simulink model "SVPWM_modified_working"  (R2015b)
settings: Solver=VariableStepAuto  StartTime=0.0  StopTime=0.1  RelTol=1e-3
libraries: powerlib x33, simulink x7
settings Model: Creator=hakan  LastModifiedBy=hakan

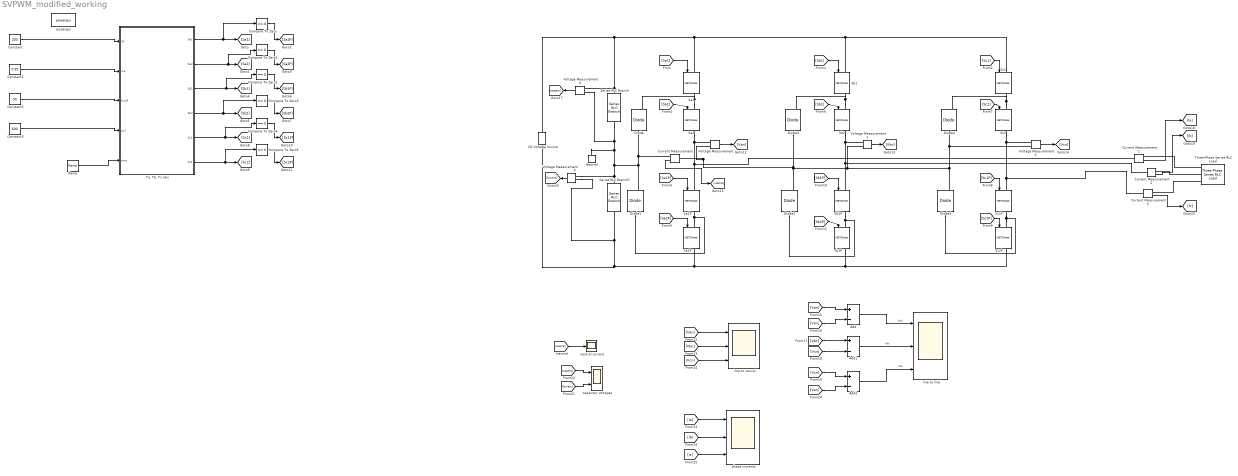
== system SVPWM_modified_working ==
  Add : Sum  Inputs=+-
  Add1 : Sum  Inputs=+-
  Add2 : Sum  Inputs=+-
  Compare To Zero{,1..5} (6 alike) : simulink/Logic and Bit Operations/Compare To Zero  relop===  OutDataTypeStr=boolean
  Constant : Constant  Value=200
  Constant1 : Constant  Value=0.95
  Constant2 : Constant  Value=50
  Constant3 : Constant  Value=600  VectorParams1D=off
  Current Measurement{,1..3} (4 alike) : powerlib/Measurements/Current Measurement  PhasorSimulation=off  OutputType=Complex  PSBequivalent=0
  DC Voltage Source : powerlib/Electrical Sources/DC Voltage Source  Amplitude=540  Measurements=None
  Diode{,1..5} (6 alike) : powerlib/Power Electronics/Diode  Ron=0.001  Lon=0  Vf=0.8  IC=0  UseSnubber=off  Rs=500  Cs=250e-9  Measurements=on
  Neutral : powerlib/Elements/Neutral  LConnTagsString=a  NodeNumber=10
  Ramp : simulink/Sources/Ramp  slope=1  start=0  X0=0
  "Sa1 " : powerlib/Power Electronics/IGBT//Diode  Ron=1e-3  Rs=1e5  Cs=inf  Measurements=on
  Sa1P : powerlib/Power Electronics/IGBT//Diode  Ron=1e-3  Rs=1e5  Cs=inf  Measurements=on
  Sa2 : powerlib/Power Electronics/IGBT//Diode  Ron=1e-3  Rs=1e5  Cs=inf  Measurements=on
  Sa2P : powerlib/Power Electronics/IGBT//Diode  Ron=1e-3  Rs=1e5  Cs=inf  Measurements=on
  Sb1 : powerlib/Power Electronics/IGBT//Diode  Ron=1e-3  Rs=1e5  Cs=inf  Measurements=on
  Sb1P : powerlib/Power Electronics/IGBT//Diode  Ron=1e-3  Rs=1e5  Cs=inf  Measurements=on
  Sb2 : powerlib/Power Electronics/IGBT//Diode  Ron=1e-3  Rs=1e5  Cs=inf  Measurements=on
  Sb2P : powerlib/Power Electronics/IGBT//Diode  Ron=1e-3  Rs=1e5  Cs=inf  Measurements=on
  Sc1 : powerlib/Power Electronics/IGBT//Diode  Ron=1e-3  Rs=1e5  Cs=inf  Measurements=on
  Sc1P : powerlib/Power Electronics/IGBT//Diode  Ron=1e-3  Rs=1e5  Cs=inf  Measurements=on
  Sc2 : powerlib/Power Electronics/IGBT//Diode  Ron=1e-3  Rs=1e5  Cs=inf  Measurements=on
  Sc2P : powerlib/Power Electronics/IGBT//Diode  Ron=1e-3  Rs=1e5  Cs=inf  Measurements=on
  Series RLC Branch : powerlib/Elements/Series RLC Branch  LConnTagsString=__new0  RConnTagsString=__new0  BranchType=RC  Resistance=1  Inductance=1e-3  SetiL0=off  InitialCurrent=0  Capacitance=1000e-6  Setx0=off  InitialVoltage=0  Measurements=None
  Series RLC Branch1 : powerlib/Elements/Series RLC Branch  LConnTagsString=__new0  RConnTagsString=__new0  BranchType=RC  Resistance=1  Inductance=1e-3  SetiL0=off  InitialCurrent=0  Capacitance=1000e-6  Setx0=off  InitialVoltage=0  Measurements=None
  "Ta, Tb, Tc calc" : MATLAB Function  TreatAsAtomicUnit=on
  Three-Phase Series RLC Load : powerlib/Elements/Three-Phase Series RLC Load  LConnTagsString=A|B|C  Configuration=Y (grounded)  NominalVoltage=1000  Vabc=[1e3 1e3 1e3]  Vabcp=[1e3 1e3 1e3]  NominalFrequency=50  UnbalancedPower=off  ActivePower=10000  InductivePower=4000  CapacitivePower=0  Pabc=[10e3 9e3 11e3]  QLabc=[100 90 110]  QCabc=[100 90 110]  Pabcp=[10e3 9e3 11e3]  QLabcp=[100 90 110]  QCabcp=[100 90 110]  Measurements=None  LoadType=constant Z
  Voltage Measurement{,1..4} (5 alike) : powerlib/Measurements/Voltage Measurement  PhasorSimulation=off  OutputType=Complex  PSBequivalent=0
  capacitor voltages : Scope  NumInputPorts=2
  line to line : Scope  NumInputPorts=3
  line to neural : Scope  NumInputPorts=3
  neutral current : Scope
  phase currents : Scope  NumInputPorts=3
  powergui : powerlib/powergui  Priority=1  SimulationMode=Continuous  SolverType=Tustin/Backward Euler (TBE)  SampleTime=50e-6  frequency=60  SPID=off  DisableSnubberDevices=off  DisableRonSwitches=off  DisableVfSwitches=off  SwTol=0  DisplayEquations=off  Interpol=off  ExternalGateDelay=off  methode=off  Ts=10  FunctionMessages=off  echomessages=off  HookPort=off  EnableUseOfTLC=off  x0status=blocks  frequencyindice=0  Pbase=100e6  ErrMax=1e-4  Iterations=50  UnitsV=kV  UnitsW=MW  buscounter=0  RestoreLinks=warning  ResistiveCurrentMeasurement=off  Frange=[0:2:500]  Ylog=off  Xlog=on  ShowGrid=off  save=off  variable=ZData  structure=linetoline  ZoomFFT=off  StartTime=0.0  cycles=2  DisplayStyle=1  fundamental=50  FreqAxis=off  MaxFrequency=5000  frequencyindicesteady=1  RmsSteady=1  display=off
  wires:
  Constant/1 -> "Ta, Tb, Tc calc"/1(Vd)
  Constant1/1 -> "Ta, Tb, Tc calc"/2(ma)
  Constant2/1 -> "Ta, Tb, Tc calc"/3(fundf)
  Constant3/1 -> "Ta, Tb, Tc calc"/4(swf)
  "Ta, Tb, Tc calc"/1(Sa1) -> Compare To Zero/1, [Sa1]
  "Ta, Tb, Tc calc"/2(Sa2) -> Compare To Zero1/1, [Sa2]
  "Ta, Tb, Tc calc"/3(Sb1) -> Compare To Zero2/1, [Sb1]
  "Ta, Tb, Tc calc"/4(Sb2) -> Compare To Zero3/1, [Sb2]
  "Ta, Tb, Tc calc"/5(Sc1) -> Compare To Zero4/1, [Sc1]
  "Ta, Tb, Tc calc"/6(Sc2) -> Compare To Zero5/1, [Sc2]
  Compare To Zero/1 -> [Sa1P]
  Compare To Zero1/1 -> [Sa2P]
  Compare To Zero2/1 -> [Sb1P]
  Compare To Zero3/1 -> [Sb2P]
  Compare To Zero4/1 -> [Sc1P]
  Compare To Zero5/1 -> [Sc2P]
  [Sa1] -> "Sa1 "/1
  [Sa1P] -> Sa1P/1
  [Sa2] -> Sa2/1
  [Sa2P] -> Sa2P/1
  [Sb1] -> Sb1/1
  [Sb2] -> Sb2/1
  [Sb1P] -> Sb1P/1
  [Sb2P] -> Sb2P/1
  [Sc2P] -> Sc2P/1
  [Sc1P] -> Sc1P/1
  [Sc1] -> Sc1/1
  [Sc2] -> Sc2/1
  Ramp/1 -> "Ta, Tb, Tc calc"/5(time)
  Voltage Measurement/1 -> [Van]
  Voltage Measurement1/1 -> [Vbn]
  Voltage Measurement2/1 -> [Vcn]
  [Van] -> line to neural/1
  [Vbn] -> line to neural/2
  [Vcn] -> line to neural/3
  [Van] -> Add/1
  [Vbn] -> Add/2
  Add/1 -> line to line/1  "Vab"
  [Vbn] -> Add1/1
  [Vcn] -> Add1/2
  Add1/1 -> line to line/2  "Vbc"
  [Vcn] -> Add2/1
  [Van] -> Add2/2
  Add2/1 -> line to line/3  "Vca"
  Current Measurement/1 -> [Ineutral]
  [Ineutral] -> neutral current/1
  Voltage Measurement3/1 -> [lowerc]
  [lowerc] -> capacitor voltages/2
  Voltage Measurement4/1 -> [upperc]
  [upperc] -> capacitor voltages/1
  Current Measurement1/1 -> [Ia]
  Current Measurement2/1 -> [Ib]
  Current Measurement3/1 -> [Ic]
  [Ib] -> phase currents/2
  [Ia] -> phase currents/1
  [Ic] -> phase currents/3
  connections:
  DC Voltage Source/RConn1 -- Sc1/LConn1 -- Sb1/LConn1 -- "Sa1 "/LConn1 -- Voltage Measurement4/LConn1 -- Series RLC Branch/LConn1
  DC Voltage Source/LConn1 -- Sb2P/RConn1 -- Sc2P/RConn1 -- Sa2P/RConn1 -- Voltage Measurement3/LConn2 -- Series RLC Branch1/RConn1
  Sa2/LConn1 -- "Sa1 "/RConn1 -- Diode/RConn1
  Sa2/RConn1 -- Current Measurement1/LConn1 -- Sa1P/LConn1 -- Voltage Measurement/LConn1
  Sa2P/LConn1 -- Sa1P/RConn1 -- Diode1/LConn1
  Sb2/LConn1 -- Sb1/RConn1 -- Diode3/RConn1
  Sb2/RConn1 -- Sb1P/LConn1 -- Current Measurement2/LConn1 -- Voltage Measurement1/LConn1
  Sb2P/LConn1 -- Sb1P/RConn1 -- Diode2/LConn1
  Sc2/LConn1 -- Sc1/RConn1 -- Diode4/RConn1
  Sc2/RConn1 -- Voltage Measurement2/LConn1 -- Current Measurement3/LConn1 -- Sc1P/LConn1
  Sc2P/LConn1 -- Sc1P/RConn1 -- Diode5/LConn1
  Diode3/LConn1 -- Voltage Measurement/LConn2 -- Current Measurement/LConn1 -- Voltage Measurement2/LConn2 -- Diode4/LConn1 -- Diode5/RConn1 -- Voltage Measurement1/LConn2 -- Diode2/RConn1
  Series RLC Branch/RConn1 -- Voltage Measurement4/LConn2 -- Voltage Measurement3/LConn1 -- Series RLC Branch1/LConn1 -- Current Measurement/RConn1 -- Diode/LConn1 -- Diode1/RConn1 -- Neutral/LConn1
  Three-Phase Series RLC Load/LConn1 -- Current Measurement1/RConn1
  Three-Phase Series RLC Load/LConn2 -- Current Measurement2/RConn1
  Three-Phase Series RLC Load/LConn3 -- Current Measurement3/RConn1

== matlab function SVPWM_modified_working/Ta, Tb, Tc calc ==
  data: Sa1 output; Sa2 output; Sb1 output; Sb2 output; Vd input; ma input; fundf input; swf input; time input; Sc1 output; Sc2 output
function [Sa1, Sa2, Sb1, Sb2, Sc1, Sc2] = fcn(Vd,ma,fundf, swf, time)
% this program works for magnitude of Vref is greater then Vd/3 meaning ma
% must be greater than 1/sqrt(3). for smaller ma's computation is a bit
% more tricky therefore it is omitted for simplicity for now. 
%#ok<*NASGU>
Vref = ma*Vd/sqrt(3); %magnitude of Vref
theta = 2*pi*fundf*time; %angle of Vref
angle = mod(theta, 2*pi);
Ts = 1/swf;
Ta = 0;
Tb = 0;
Tc = 0;
output = 0;
Sector1 = 0; Sector2 = 0; Sector3 = 0; Sector4= 0; Sector5 = 0; Sector6 = 0;
rgn2a = 0 ;rgn2b = 0; rgn3 = 0; rgn4 = 0;
Sa1=0; Sa2=0; Sa1P=0; Sa2P=0; Sb1=0; Sb2=0; Sb1P=0; Sb2P=0; Sc1=0; Sc2=0; Sc1P=0; Sc2P=0;
anglefrom3to2= 0 ;
timee = mod(time, Ts);

%% Sector 1


if (mod(theta, 2*pi)<=pi/3)&&(mod(theta, 2*pi)>0)  % sector 1

    n = 1;
    thetaprime = angle - (n-1)*pi/3;
        for aci = 0:0.00001:pi/3   
            la = sqrt(3)*cos(aci)-sin(aci);
                if (la*ma > 0.99)&&(la*ma<=1)
                    anglefrom3to2 = aci; %leaving angle from region 3 to region 2
                    break
                end
        end

    %anglefrom3to2 = asin(1-1/(sqrt(3)*ma)); 
    anglefrom2to4 = pi/3 - anglefrom3to2; %leaving angle from region 2 to region 4
    if (mod(theta, 2*pi)<=anglefrom3to2) % then sector 1 region 3
        rgn2a = 0 ;rgn2b = 0; rgn3 = 1; rgn4 = 0;
        Ta = Ts*(2-2*ma*sin(pi/3+thetaprime));
        Tb = Ts*2*ma*sin(thetaprime);
        Tc = Ts*(2*ma*sin(pi/3-thetaprime)-1);  
        times = [Tc/4 Tb/2 Ta/2 Tc/2 Ta/2 Tb/2 Tc/4];
        times = cumsum(times);
        va1 = [1 1 1 0 1 1 1];
        va2 = [1 1 1 1 1 1 1];
        vb1 = [0 0 0 0 0 0 0];
        vb2 = [1 1 0 0 0 1 1];
        vc1 = [0 0 0 0 0 0 0];
        vc2 = [1 0 0 0 0 0 1];
        for j = 1:7
            
            if(timee<times(j))
                break
            end
        end
        Sa1=va1(j); Sa2=va2(j);
        Sb1=vb1(j); Sb2=vb2(j); 
        Sc1=vc1(j); Sc2=vc2(j); 
    else if (mod(theta,2*pi)>anglefrom3to2)&&(mod(theta,2*pi)<=anglefrom2to4) % then sector 1 region 2
            if angle<= pi/6 % then 2a
                rgn2a= 1; rgn2b = 0; rgn3 = 0; rgn4=0;
            else % then 2b
                rgn2a= 0; rgn2b = 1; rgn3 = 0; rgn4=0;
            end
            Ta = Ts*(1-2*ma*sin(thetaprime));
            Tb = Ts*(2*ma*sin(pi/3+thetaprime)-1);
            Tc = Ts*(1-2*ma*sin(pi/3-thetaprime));  
            times = [Tc/4 Tb/2 Ta/2 Tc/2 Ta/2 Tb/2 Tc/4];
            times = cumsum(times);
        if(rgn2a)
            va1 = [1 1 0 0 0 1 1];
            va2 = [1 1 1 1 1 1 1];
            vb1 = [0 0 0 0 0 0 0];
            vb2 = [1 1 1 0 1 1 1];
            vc1 = [0 0 0 0 0 0 0];
            vc2 = [1 0 0 0 0 0 1];
        for j = 1:7
            if(timee<times(j))
                break
            end
        end
        Sa1=va1(j); Sa2=va2(j);
        Sb1=vb1(j); Sb2=vb2(j); 
        Sc1=vc1(j); Sc2=vc2(j); 
        end
        if(rgn2b)
            va1 = [0 1 1 1 1 1 0];
            va2 = [1 1 1 1 1 1 1];
            vb1 = [0 0 0 1 0 0 0];
            vb2 = [1 1 1 1 1 1 1];
            vc1 = [0 0 0 0 0 0 0];
            vc2 = [0 0 1 1 1 0 0];
        for j = 1:7
            if(timee<times(j))
                break
            end
        end
        Sa1=va1(j); Sa2=va2(j);
        Sb1=vb1(j); Sb2=vb2(j); 
        Sc1=vc1(j); Sc2=vc2(j);     
        end
            
        else if (mod(theta,2*pi)>anglefrom2to4) % then sector 1 region 4
               rgn2a = 0 ;rgn2b = 0; rgn3 = 0; rgn4 = 1;
               Ta = Ts*(2*ma*sin(thetaprime)-1);
               Tb = Ts*(2*ma*sin(pi/3-thetaprime));
               Tc = Ts*(2-2*ma*sin(pi/3+thetaprime));  
               times = [Tc/4 Tb/2 Ta/2 Tc/2 Ta/2 Tb/2 Tc/4];
               times = cumsum(times);
        va1 = [0 1 1 1 1 1 0];
        va2 = [1 1 1 1 1 1 1];
        vb1 = [0 0 1 1 1 0 0];
        vb2 = [1 1 1 1 1 1 1];
        vc1 = [0 0 0 0 0 0 0];
        vc2 = [0 0 0 1 0 0 0];
        for j = 1:7
            if(timee<times(j))
                break
            end
        end
        Sa1=va1(j); Sa2=va2(j);
        Sb1=vb1(j); Sb2=vb2(j); 
        Sc1=vc1(j); Sc2=vc2(j);
            end
        end
    end
    Sector1 = 1; Sector2 = 0; Sector3 = 0; Sector4= 0; Sector5 = 0; Sector6 = 0;
end
%% Sector 2


if (mod(theta, 2*pi)<=2*pi/3)&&(mod(theta, 2*pi)>pi/3)  % sector 2
    
    n = 2;
    thetaprime = angle - (n-1)*pi/3;
        for aci = 0:0.00001:pi/3   
            la = sqrt(3)*cos(aci)-sin(aci);
                if (la*ma > 0.99)&&(la*ma<=1)
                    anglefrom3to2 = aci+pi/3; %leaving angle from region 3 to region 2
                    break
                end
        end
    %anglefrom3to2 = pi/3 + asin(1-1/(sqrt(3)*ma));
    anglefrom2to4 = pi/3 + pi/3 - anglefrom3to2;
    if (mod(theta, 2*pi)<=anglefrom3to2) % then sector 2 region 3
        rgn2a = 0 ;rgn2b = 0; rgn3 = 1; rgn4 = 0;
        Ta = Ts*(2-2*ma*sin(pi/3+thetaprime));
        Tb = Ts*2*ma*sin(thetaprime);
        Tc = Ts*(2*ma*sin(pi/3-thetaprime)-1);
        times = [Tc/4 Tb/2 Ta/2 Tc/2 Ta/2 Tb/2 Tc/4];
        times = cumsum(times);
        va1 = [0 0 1 1 1 0 0];
        va2 = [1 1 1 1 1 1 1];
        vb1 = [0 1 1 1 1 1 0];
        vb2 = [1 1 1 1 1 1 1];
        vc1 = [0 0 0 0 0 0 0];
        vc2 = [0 0 0 1 0 0 0];
        for j = 1:7
            if(timee<times(j))
                break
            end
        end
        Sa1=va1(j); Sa2=va2(j);
        Sb1=vb1(j); Sb2=vb2(j); 
        Sc1=vc1(j); Sc2=vc2(j);
    else if (mod(theta,2*pi)>anglefrom3to2)&&(mod(theta,2*pi)<=anglefrom2to4) % then sector 2 region 2
            if angle<=pi/2 %then 2a
                rgn2a= 1; rgn2b = 0; rgn3 = 0; rgn4=0;
            else % then 2b
                rgn2a= 0; rgn2b = 1; rgn3 = 0; rgn4=0;
            end
            Ta = Ts*(1-2*ma*sin(thetaprime));
            Tb = Ts*(2*ma*sin(pi/3+thetaprime)-1);
            Tc = Ts*(1-2*ma*sin(pi/3-thetaprime)); 
            times = [Tc/4 Tb/2 Ta/2 Tc/2 Ta/2 Tb/2 Tc/4];
            times = cumsum(times);
        if(rgn2a)
            va1 = [0 0 0 1 0 0 0];
            va2 = [1 1 1 1 1 1 1];
            vb1 = [0 1 1 1 1 1 0];
            vb2 = [1 1 1 1 1 1 1];
            vc1 = [0 0 0 0 0 0 0];
            vc2 = [0 0 1 1 1 0 0];
        for j = 1:7
            if(timee<times(j))
                break
            end
        end
        Sa1=va1(j); Sa2=va2(j);
        Sb1=vb1(j); Sb2=vb2(j); 
        Sc1=vc1(j); Sc2=vc2(j); 
        end
        if(rgn2b)
            va1 = [0 0 0 0 0 0 0];
            va2 = [1 1 1 0 1 1 1];
            vb1 = [1 1 0 0 0 1 1];
            vb2 = [1 1 1 1 1 1 1];
            vc1 = [0 0 0 0 0 0 0];
            vc2 = [1 0 0 0 0 0 1];
        for j = 1:7
            if(timee<times(j))
                break
            end
        end
        Sa1=va1(j); Sa2=va2(j);
        Sb1=vb1(j); Sb2=vb2(j); 
        Sc1=vc1(j); Sc2=vc2(j);     
        end
        else if (mod(theta,2*pi)>anglefrom2to4) % then sector 2 region 4
               rgn2a = 0 ;rgn2b = 0; rgn3 = 0; rgn4 = 1;
               Ta = Ts*(2*ma*sin(thetaprime)-1);
               Tb = Ts*(2*ma*sin(pi/3-thetaprime));
               Tc = Ts*(2-2*ma*sin(pi/3+thetaprime));
               times = [Tc/4 Tb/2 Ta/2 Tc/2 Ta/2 Tb/2 Tc/4];
               times = cumsum(times);
        va1 = [0 0 0 0 0 0 0];
        va2 = [1 1 0 0 0 1 1];
        vb1 = [1 1 1 0 1 1 1];
        vb2 = [1 1 1 1 1 1 1];
        vc1 = [0 0 0 0 0 0 0];
        vc2 = [1 0 0 0 0 0 1];
        for j = 1:7
            if(timee<times(j))
                break
            end
        end
        Sa1=va1(j); Sa2=va2(j);
        Sb1=vb1(j); Sb2=vb2(j); 
        Sc1=vc1(j); Sc2=vc2(j);
            end
        end
    end
    Sector1 = 0; Sector2 = 1; Sector3 = 0; Sector4= 0; Sector5 = 0; Sector6 = 0;
end
%% Sector 3

if (mod(theta, 2*pi)<=pi)&&(mod(theta, 2*pi)>2*pi/3)  % sector 3
    
    n = 3;
    thetaprime = angle - (n-1)*pi/3;
        for aci = 0:0.00001:pi/3   
            la = sqrt(3)*cos(aci)-sin(aci);
                if (la*ma > 0.99)&&(la*ma<=1)
                    anglefrom3to2 = aci+pi/3+pi/3; %leaving angle from region 3 to region 2
                    break
                end
        end    
    %anglefrom3to2 = 2*pi/3 + asin(1-1/(sqrt(3)*ma));
    anglefrom2to4 = 2*pi/3 + pi/3 - anglefrom3to2;
    if (mod(theta, 2*pi)<=anglefrom3to2) % then sector 3 region 3
        rgn2a = 0 ;rgn2b = 0; rgn3 = 1; rgn4 = 0;
        Ta = Ts*(2-2*ma*sin(pi/3+thetaprime));
        Tb = Ts*2*ma*sin(thetaprime);
        Tc = Ts*(2*ma*sin(pi/3-thetaprime)-1); 
        times = [Tc/4 Tb/2 Ta/2 Tc/2 Ta/2 Tb/2 Tc/4];
        times = cumsum(times);
        va1 = [0 0 0 0 0 0 0];
        va2 = [1 0 0 0 0 0 1];
        vb1 = [1 1 1 0 1 1 1];
        vb2 = [1 1 1 1 1 1 1];
        vc1 = [0 0 0 0 0 0 0];
        vc2 = [1 1 0 0 0 1 1];
        for j = 1:7
            if(timee<times(j))
                break
            end
        end
        Sa1=va1(j); Sa2=va2(j);
        Sb1=vb1(j); Sb2=vb2(j); 
        Sc1=vc1(j); Sc2=vc2(j);
    else if (mod(theta,2*pi)>anglefrom3to2)&&(mod(theta,2*pi)<=anglefrom2to4) % then sector 3 region 2
            if angle<=5*pi/6 %then 2a
                rgn2a= 1; rgn2b = 0; rgn3 = 0; rgn4=0;
            else % then 2b
                rgn2a= 0; rgn2b = 1; rgn3 = 0; rgn4=0;
            end
            Ta = Ts*(1-2*ma*sin(thetaprime));
            Tb = Ts*(2*ma*sin(pi/3+thetaprime)-1);
            Tc = Ts*(1-2*ma*sin(pi/3-thetaprime));
            times = [Tc/4 Tb/2 Ta/2 Tc/2 Ta/2 Tb/2 Tc/4];
            times = cumsum(times);
            if(rgn2a)
            va1 = [0 0 0 0 0 0 0];
            va2 = [1 0 0 0 0 0 1];
            vb1 = [1 1 0 0 0 1 1];
            vb2 = [1 1 1 1 1 1 1];
            vc1 = [0 0 0 0 0 0 0];
            vc2 = [1 1 1 0 1 1 1];
        for j = 1:7
            if(timee<times(j))
                break
            end
        end
        Sa1=va1(j); Sa2=va2(j);
        Sb1=vb1(j); Sb2=vb2(j); 
        Sc1=vc1(j); Sc2=vc2(j); 
        end
        if(rgn2b)
            va1 = [0 0 0 0 0 0 0];
            va2 = [0 0 1 1 1 0 0];
            vb1 = [0 1 1 1 1 1 0];
            vb2 = [1 1 1 1 1 1 1];
            vc1 = [0 0 0 1 0 0 0];
            vc2 = [1 1 1 1 1 1 1];
        for j = 1:7
            if(timee<times(j))
                break
            end
        end
        Sa1=va1(j); Sa2=va2(j);
        Sb1=vb1(j); Sb2=vb2(j); 
        Sc1=vc1(j); Sc2=vc2(j);     
        end
        else if (mod(theta,2*pi)>anglefrom2to4) % then sector 3 region 4
                rgn2a = 0 ;rgn2b = 0; rgn3 = 0; rgn4 = 1;
               Ta = Ts*(2*ma*sin(thetaprime)-1);
               Tb = Ts*(2*ma*sin(pi/3-thetaprime));
               Tc = Ts*(2-2*ma*sin(pi/3+thetaprime));
               times = [Tc/4 Tb/2 Ta/2 Tc/2 Ta/2 Tb/2 Tc/4];
               times = cumsum(times);
        va1 = [0 0 0 0 0 0 0];
        va2 = [0 0 0 1 0 0 0];
        vb1 = [0 1 1 1 1 1 0];
        vb2 = [1 1 1 1 1 1 1];
        vc1 = [0 0 1 1 1 0 0];
        vc2 = [1 1 1 1 1 1 1];
        for j = 1:7
            if(timee<times(j))
                break
            end
        end
        Sa1=va1(j); Sa2=va2(j);
        Sb1=vb1(j); Sb2=vb2(j); 
        Sc1=vc1(j); Sc2=vc2(j);
            end
        end
    end
    Sector1 = 0; Sector2 = 0; Sector3 = 1; Sector4= 0; Sector5 = 0; Sector6 = 0;
end

%% Sector 4


if (mod(theta, 2*pi)<=4*pi/3)&&(mod(theta, 2*pi)>pi)  % sector 4
    

    n = 4;
    thetaprime = angle - (n-1)*pi/3;
        for aci = 0:0.00001:pi/3   
            la = sqrt(3)*cos(aci)-sin(aci);
                if (la*ma > 0.99)&&(la*ma<=1)
                    anglefrom3to2 = aci+pi/3+pi/3+pi/3; %leaving angle from region 3 to region 2
                    break
                end
        end    
    %anglefrom3to2 = pi + asin(1-1/(sqrt(3)*ma));
    anglefrom2to4 = pi + pi/3 - anglefrom3to2;
    if (mod(theta, 2*pi)<=anglefrom3to2) % then sector 4 region 3
        rgn2a = 0 ;rgn2b = 0; rgn3 = 1; rgn4 = 0;
        Ta = Ts*(2-2*ma*sin(pi/3+thetaprime));
        Tb = Ts*2*ma*sin(thetaprime);
        Tc = Ts*(2*ma*sin(pi/3-thetaprime)-1);
        times = [Tc/4 Tb/2 Ta/2 Tc/2 Ta/2 Tb/2 Tc/4];
        times = cumsum(times);
        va1 = [0 0 0 0 0 0 0];
        va2 = [0 0 0 1 0 0 0];
        vb1 = [0 0 1 1 1 0 0];
        vb2 = [1 1 1 1 1 1 1];
        vc1 = [0 1 1 1 1 1 0];
        vc2 = [1 1 1 1 1 1 1];
        for j = 1:7
            if(timee<times(j))
                break
            end
        end
        Sa1=va1(j); Sa2=va2(j);
        Sb1=vb1(j); Sb2=vb2(j); 
        Sc1=vc1(j); Sc2=vc2(j);
    else if (mod(theta,2*pi)>anglefrom3to2)&&(mod(theta,2*pi)<=anglefrom2to4) % then sector 4 region 2
            if angle<=7*pi/6 %then 2a
                rgn2a= 1; rgn2b = 0; rgn3 = 0; rgn4=0;
            else % then 2b
                rgn2a= 0; rgn2b = 1; rgn3 = 0; rgn4=0;
            end
            Ta = Ts*(1-2*ma*sin(thetaprime));
            Tb = Ts*(2*ma*sin(pi/3+thetaprime)-1);
            Tc = Ts*(1-2*ma*sin(pi/3-thetaprime));
            times = [Tc/4 Tb/2 Ta/2 Tc/2 Ta/2 Tb/2 Tc/4];
            times = cumsum(times);
             if(rgn2a)
            va1 = [0 0 0 0 0 0 0];
            va2 = [0 0 1 1 1 0 0];
            vb1 = [0 0 0 1 0 0 0];
            vb2 = [1 1 1 1 1 1 1];
            vc1 = [0 1 1 1 1 1 0];
            vc2 = [1 1 1 1 1 1 1];
        for j = 1:7
            if(timee<times(j))
                break
            end
        end
        Sa1=va1(j); Sa2=va2(j);
        Sb1=vb1(j); Sb2=vb2(j); 
        Sc1=vc1(j); Sc2=vc2(j); 
        end
        if(rgn2b)
            va1 = [0 0 0 0 0 0 0];
            va2 = [1 0 0 0 0 0 1];
            vb1 = [0 0 0 0 0 0 0];
            vb2 = [1 1 1 0 1 1 1];
            vc1 = [1 1 0 0 0 1 1];
            vc2 = [1 1 1 1 1 1 1];
        for j = 1:7
            if(timee<times(j))
                break
            end
        end
        Sa1=va1(j); Sa2=va2(j);
        Sb1=vb1(j); Sb2=vb2(j); 
        Sc1=vc1(j); Sc2=vc2(j);     
        end
        else if (mod(theta,2*pi)>anglefrom2to4) % then sector 4 region 4
                rgn2a = 0 ;rgn2b = 0; rgn3 = 0; rgn4 = 1;
               Ta = Ts*(2*ma*sin(thetaprime)-1);
               Tb = Ts*(2*ma*sin(pi/3-thetaprime));
               Tc = Ts*(2-2*ma*sin(pi/3+thetaprime));
               times = [Tc/4 Tb/2 Ta/2 Tc/2 Ta/2 Tb/2 Tc/4];
               times = cumsum(times);
               va1 = [0 0 0 0 0 0 0];
        va2 = [1 0 0 0 0 0 1];
        vb1 = [0 0 0 0 0 0 0];
        vb2 = [1 1 0 0 0 1 1];
        vc1 = [1 1 1 0 1 1 1];
        vc2 = [1 1 1 1 1 1 1];
        for j = 1:7
            if(timee<times(j))
                break
            end
        end
        Sa1=va1(j); Sa2=va2(j);
        Sb1=vb1(j); Sb2=vb2(j); 
        Sc1=vc1(j); Sc2=vc2(j);
            end
        end
    end
    Sector1 = 0; Sector2 = 0; Sector3 = 0; Sector4= 1; Sector5 = 0; Sector6 = 0;
end
%% Sector 5 

if (mod(theta, 2*pi)<=5*pi/3)&&(mod(theta, 2*pi)>4*pi/3)  % sector 5
    
    n = 5;
    thetaprime = angle - (n-1)*pi/3;
    %anglefrom3to2 = 4*pi/3 + asin(1-1/(sqrt(3)*ma));
        for aci = 0:0.00001:pi/3   
            la = sqrt(3)*cos(aci)-sin(aci);
                if (la*ma > 0.99)&&(la*ma<=1)
                    anglefrom3to2 = aci+pi/3+pi/3+pi/3+pi/3; %leaving angle from region 3 to region 2
                    break
                end
        end    
    anglefrom2to4 = 4*pi/3 + pi/3 - anglefrom3to2;
    if (mod(theta, 2*pi)<=anglefrom3to2) % then sector 5 region 3
        rgn2a = 0 ;rgn2b = 0; rgn3 = 1; rgn4 = 0;
        Ta = Ts*(2-2*ma*sin(pi/3+thetaprime));
        Tb = Ts*2*ma*sin(thetaprime);
        Tc = Ts*(2*ma*sin(pi/3-thetaprime)-1);
        times = [Tc/4 Tb/2 Ta/2 Tc/2 Ta/2 Tb/2 Tc/4];
            times = cumsum(times);
            va1 = [0 0 0 0 0 0 0];
        va2 = [1 1 0 0 0 1 1];
        vb1 = [0 0 0 0 0 0 0];
        vb2 = [1 0 0 0 0 0 1];
        vc1 = [1 1 1 0 1 1 1];
        vc2 = [1 1 1 1 1 1 1];
        for j = 1:7
            if(timee<times(j))
                break
            end
        end
        Sa1=va1(j); Sa2=va2(j);
        Sb1=vb1(j); Sb2=vb2(j); 
        Sc1=vc1(j); Sc2=vc2(j);
    else if (mod(theta,2*pi)>anglefrom3to2)&&(mod(theta,2*pi)<=anglefrom2to4) % then sector 5 region 2
            if angle<=3*pi/2 %then 2a
                rgn2a= 1; rgn2b = 0; rgn3 = 0; rgn4=0;
            else % then 2b
                rgn2a= 0; rgn2b = 1; rgn3 = 0; rgn4=0;
            end
            Ta = Ts*(1-2*ma*sin(thetaprime));
            Tb = Ts*(2*ma*sin(pi/3+thetaprime)-1);
            Tc = Ts*(1-2*ma*sin(pi/3-thetaprime));
            times = [Tc/4 Tb/2 Ta/2 Tc/2 Ta/2 Tb/2 Tc/4];
            times = cumsum(times);
            if(rgn2a)
            va1 = [0 0 0 0 0 0 0];
            va2 = [1 1 1 0 1 1 1];
            vb1 = [0 0 0 0 0 0 0];
            vb2 = [1 0 0 0 0 0 1];
            vc1 = [1 1 0 0 0 1 1];
            vc2 = [1 1 1 1 1 1 1];
        for j = 1:7
            if(timee<times(j))
                break
            end
        end
        Sa1=va1(j); Sa2=va2(j);
        Sb1=vb1(j); Sb2=vb2(j); 
        Sc1=vc1(j); Sc2=vc2(j); 
        end
        if(rgn2b)
            va1 = [0 0 0 1 0 0 0];
            va2 = [1 1 1 1 1 1 1];
            vb1 = [0 0 0 0 0 0 0];
            vb2 = [0 0 1 1 1 0 0];
            vc1 = [0 1 1 1 1 1 0];
            vc2 = [1 1 1 1 1 1 1];
        for j = 1:7
            if(timee<times(j))
                break
            end
        end
        Sa1=va1(j); Sa2=va2(j);
        Sb1=vb1(j); Sb2=vb2(j); 
        Sc1=vc1(j); Sc2=vc2(j);     
        end
        else if (mod(theta,2*pi)>anglefrom2to4) % then sector 5 region 4
               rgn2a = 0 ;rgn2b = 0; rgn3 = 0; rgn4 = 1;
               Ta = Ts*(2*ma*sin(thetaprime)-1);
               Tb = Ts*(2*ma*sin(pi/3-thetaprime));
               Tc = Ts*(2-2*ma*sin(pi/3+thetaprime)); 
               times = [Tc/4 Tb/2 Ta/2 Tc/2 Ta/2 Tb/2 Tc/4];
               times = cumsum(times);
               va1 = [0 0 1 1 1 0 0];
        va2 = [1 1 1 1 1 1 1];
        vb1 = [0 0 0 0 0 0 0];
        vb2 = [0 0 0 1 0 0 0];
        vc1 = [0 1 1 1 1 1 0];
        vc2 = [1 1 1 1 1 1 1];
        for j = 1:7
            if(timee<times(j))
                break
            end
        end
        Sa1=va1(j); Sa2=va2(j);
        Sb1=vb1(j); Sb2=vb2(j); 
        Sc1=vc1(j); Sc2=vc2(j);
            end
        end
    end
    Sector1 = 0; Sector2 = 0; Sector3 = 0; Sector4= 0; Sector5 = 1; Sector6 = 0;
end

%% Sector 6 

if (mod(theta, 2*pi)<=2*pi)&&(mod(theta, 2*pi)>5*pi/3)  % sector 6
    
    n = 6;
    thetaprime = angle - (n-1)*pi/3;
        for aci = 0:0.00001:pi/3   
            la = sqrt(3)*cos(aci)-sin(aci);
                if (la*ma > 0.99)&&(la*ma<=1)
                    anglefrom3to2 = aci+pi/3+pi/3+pi/3+pi/3+pi/3; %leaving angle from region 3 to region 2
                    break
                end
        end    
    %anglefrom3to2 = 5*pi/3 + asin(1-1/(sqrt(3)*ma));
    anglefrom2to4 = 5*pi/3 + pi/3 - anglefrom3to2;
    if (mod(theta, 2*pi)<=anglefrom3to2) % then sector 6 region 3
        rgn2a = 0 ;rgn2b = 0; rgn3 = 1; rgn4 = 0;
        Ta = Ts*(2-2*ma*sin(pi/3+thetaprime));
        Tb = Ts*2*ma*sin(thetaprime);
        Tc = Ts*(2*ma*sin(pi/3-thetaprime)-1);
        times = [Tc/4 Tb/2 Ta/2 Tc/2 Ta/2 Tb/2 Tc/4];
        times = cumsum(times);
        va1 = [0 1 1 1 1 1 0];
        va2 = [1 1 1 1 1 1 1];
        vb1 = [0 0 0 0 0 0 0];
        vb2 = [0 0 0 1 0 0 0];
        vc1 = [0 0 1 1 1 0 0];
        vc2 = [1 1 1 1 1 1 1];
        for j = 1:7
            if(timee<times(j))
                break
            end
        end
        Sa1=va1(j); Sa2=va2(j);
        Sb1=vb1(j); Sb2=vb2(j); 
        Sc1=vc1(j); Sc2=vc2(j);
        
    else if (mod(theta,2*pi)>anglefrom3to2)&&(mod(theta,2*pi)<=anglefrom2to4) % then sector 6 region 2
            if angle<=11*pi/6 %then 2a
                rgn2a= 1; rgn2b = 0; rgn3 = 0; rgn4=0;
            else % then 2b
                rgn2a= 0; rgn2b = 1; rgn3 = 0; rgn4=0;
            end
            Ta = Ts*(1-2*ma*sin(thetaprime));
            Tb = Ts*(2*ma*sin(pi/3+thetaprime)-1);
            Tc = Ts*(1-2*ma*sin(pi/3-thetaprime));
            times = [Tc/4 Tb/2 Ta/2 Tc/2 Ta/2 Tb/2 Tc/4];
            times = cumsum(times);
            if(rgn2a)
            va1 = [0 1 1 1 1 1 0];
            va2 = [1 1 1 1 1 1 1];
            vb1 = [0 0 0 0 0 0 0];
            vb2 = [0 0 1 1 1 0 0];
            vc1 = [0 0 0 1 0 0 0];
            vc2 = [1 1 1 1 1 1 1];
        for j = 1:7
            if(timee<times(j))
                break
            end
        end
        Sa1=va1(j); Sa2=va2(j);
        Sb1=vb1(j); Sb2=vb2(j); 
        Sc1=vc1(j); Sc2=vc2(j); 
        end
        if(rgn2b)
            va1 = [1 1 0 0 0 1 1];
            va2 = [1 1 1 1 1 1 1];
            vb1 = [0 0 0 0 0 0 0];
            vb2 = [1 0 0 0 0 0 1];
            vc1 = [0 0 0 0 0 0 0];
            vc2 = [1 1 1 0 1 1 1];
        for j = 1:7
            if(timee<times(j))
                break
            end
        end
        Sa1=va1(j); Sa2=va2(j);
        Sb1=vb1(j); Sb2=vb2(j); 
        Sc1=vc1(j); Sc2=vc2(j);     
        end
        else if (mod(theta,2*pi)>anglefrom2to4) % then sector 6 region 4
               rgn2a = 0 ;rgn2b = 0; rgn3 = 0; rgn4 = 1;
               Ta = Ts*(2*ma*sin(thetaprime)-1);
               Tb = Ts*(2*ma*sin(pi/3-thetaprime));
               Tc = Ts*(2-2*ma*sin(pi/3+thetaprime));
               times = [Tc/4 Tb/2 Ta/2 Tc/2 Ta/2 Tb/2 Tc/4];
               times = cumsum(times);
               va1 = [1 1 1 0 1 1 1];
        va2 = [1 1 1 1 1 1 1];
        vb1 = [0 0 0 0 0 0 0];
        vb2 = [1 0 0 0 0 0 1];
        vc1 = [0 0 0 0 0 0 0];
        vc2 = [1 1 0 0 0 1 1];
        for j = 1:7
            if(timee<times(j))
                break
            end
        end
        Sa1=va1(j); Sa2=va2(j);
        Sb1=vb1(j); Sb2=vb2(j); 
        Sc1=vc1(j); Sc2=vc2(j);
            end
        end
    end
    Sector1 = 0; Sector2 = 0; Sector3 = 0; Sector4= 0; Sector5 = 0; Sector6 = 1;
end
